simulink model "Mux1"  (R2024b)
settings: Solver=VariableStepAuto  StartTime=0.0  StopTime=10.0  RelTol=1e-3
settings Model: Creator=Ahmad  LastModifiedBy=Ahmad

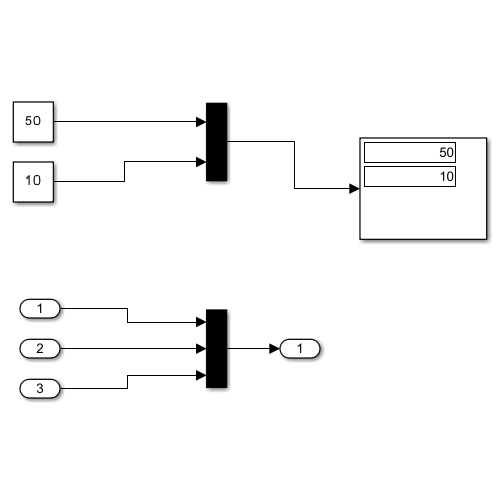
[thumbnail: Simulink's stored preview of the top-level diagram]
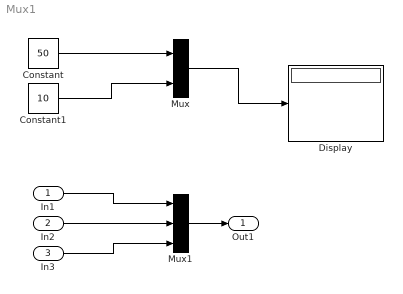
== system Mux1 ==
  In1 : Inport
  In2 : Inport  Port=2
  In3 : Inport  Port=3
  Constant : Constant  Value=50
  Constant1 : Constant  Value=10
  Display : Display
  Mux : Mux  Inputs=2
  Mux1 : Mux  Inputs=3
  Out1 : Outport
  wires:
  Constant/1 -> Mux/1
  Constant1/1 -> Mux/2
  Mux/1 -> Display/1
  In1/1 -> Mux1/1
  In2/1 -> Mux1/2
  In3/1 -> Mux1/3
  Mux1/1 -> Out1/1
